simulink model "QuadRotor_PID_Simulink3d"  (R2014a)
settings: Solver=ode45  StartTime=0.0  StopTime=inf
PreLoadFcn:
  | load CommandsBus
model workspace (MAT data in the model file):
  MCOS : class17 (value not decoded)
  MCOS : class17 (value not decoded)
undefined symbols (not defined in the file or in its folder): X, Y, Z
libraries: sm_lib x829, nesl_utility x156, simulink x12, fl_lib x4, vrlib x4, aerolibtransform2 x1
(part 15 of 18)

== system QuadRotor_PID_Simulink3d/quadSimulation/Plant_Quad_Base/Quad_Yaw_Altitude/QuadRotor/P2/MotorA ==
  SpdMotor : Inport
  External Force and Torque : sm_lib/Forces and Torques/External Force and Torque  ForceResolutionFrame=AttachedFrame  EnableForceX=off  EnableForceY=off  EnableForceZ=on  EnableForce=off  TorqueResolutionFrame=AttachedFrame  EnableTorqueX=off  EnableTorqueY=off  EnableTorqueZ=on  EnableTorque=off  BlockFunction=simmechanics.library.forces_torques.external_force_torque
  Helice_1_RIGID : Subsystem
  PS-Simulink Converter : nesl_utility/PS-Simulink Converter  PhysicalDomain=network_engine_domain  SubClassName=ps_output  LeftPortType=input  RightPortType=output  PseudoPeriodic=off  Frequencies=[]  Unit=1  AffineConversion=off
  ReferenceFrame : sm_lib/Frames and Transforms/Reference Frame  BlockFunction=simmechanics.library.frames_transforms.reference_frame
  RevPropeller : sm_lib/Joints/Revolute Joint  SenseConstraintForce=off  SenseConstraintForceX=off  SenseConstraintForceY=off  SenseConstraintForceZ=off  SenseConstraintTorque=off  SenseConstraintTorqueX=off  SenseConstraintTorqueY=off  SenseConstraintTorqueZ=off  SenseTotalForce=off  SenseTotalForceX=off  SenseTotalForceY=off  SenseTotalForceZ=off  SenseTotalTorque=off  SenseTotalTorqueX=off  SenseTotalTorqueY=off  SenseTotalTorqueZ=off  CompositeWrenchDir=FollowerOnBase  CompositeWrenchFrame=BaseFrame  EquilibriumPosition=0  EquilibriumPositionUnits=rad  SpringStiffness=0  SpringStiffnessUnits=m*N/rad  DampingCoefficient=0  DampingCoefficientUnits=m*s*N/rad  TorqueActuationMode=InputTorque  MotionActuationMode=ComputedMotion  SensePosition=off  SenseVelocity=on  SenseAcceleration=off  SenseTorqueForce=off  PositionTargetValue=-56.842386520865752  PositionTargetValueUnits=deg  PositionTargetSpecify=off  PositionTargetPriority=Low  VelocityTargetValue=0  VelocityTargetValueUnits=deg/s  VelocityTargetSpecify=off  VelocityTargetPriority=High  BlockFunction=simmechanics.library.joints.revolute_joint
  Simulink-PS Converter : nesl_utility/Simulink-PS Converter  PhysicalDomain=network_engine_domain  SubClassName=ps_input  LeftPortType=input  RightPortType=output  PseudoPeriodic=off  Frequencies=[]  NoiseDistribution=none  NoiseParameters=[]  Unit=1  AffineConversion=off  InputFiltering=off  SimscapeFilterOrder=1  InputFilterTimeConstant=0.001  UdotUserProvided=1
  Simulink-PS Converter2 : nesl_utility/Simulink-PS Converter  PhysicalDomain=network_engine_domain  SubClassName=ps_input  LeftPortType=input  RightPortType=output  PseudoPeriodic=off  Frequencies=[]  NoiseDistribution=none  NoiseParameters=[]  Unit=1  AffineConversion=off  InputFiltering=off  SimscapeFilterOrder=1  InputFilterTimeConstant=0.001  UdotUserProvided=1
  Simulink-PS Converter3 : nesl_utility/Simulink-PS Converter  PhysicalDomain=network_engine_domain  SubClassName=ps_input  LeftPortType=input  RightPortType=output  PseudoPeriodic=off  Frequencies=[]  NoiseDistribution=none  NoiseParameters=[]  Unit=1  AffineConversion=off  InputFiltering=off  SimscapeFilterOrder=1  InputFilterTimeConstant=0.001  UdotUserProvided=1
  Thrust : MATLAB Function  TreatAsAtomicUnit=on
  Transform : sm_lib/Frames and Transforms/Rigid Transform  TranslationMethod=None  TranslationLengthUnit=m  TranslationStandardAxis=+Z  TranslationStandardOffset=0  TranslationCartesianOffset=[0 0 0]  TranslationROffset=0  TranslationROffsetUnits=m  TranslationZOffset=0  TranslationZOffsetUnits=m  TranslationThetaOffset=0  TranslationThetaOffsetUnits=deg  RotationMethod=None  RotationAngleUnits=deg  RotationStandardAxis=+Z  RotationAngle=0  RotationArbitraryAxis=[0 0 1]  FollAlignAxisA=+X  BaseAlignAxisA=+Y  FollAlignAxisB=+Y  BaseAlignAxisB=+Z  BlockFunction=simmechanics.library.frames_transforms.rigid_transform
  Transform1 : sm_lib/Frames and Transforms/Rigid Transform  TranslationMethod=Cartesian  TranslationLengthUnit=mm  TranslationStandardAxis=+Z  TranslationStandardOffset=0  TranslationCartesianOffset=[0 25 0]  TranslationROffset=0  TranslationROffsetUnits=m  TranslationZOffset=0  TranslationZOffsetUnits=m  TranslationThetaOffset=0  TranslationThetaOffsetUnits=deg  RotationMethod=ArbitraryAxis  RotationAngleUnits=rad  RotationStandardAxis=+Z  RotationAngle=1.6523019578475986  RotationArbitraryAxis=[-0.92164420581175521 -0.27438290571172536 -0.27438290571172536]  FollAlignAxisA=+X  BaseAlignAxisA=+Y  FollAlignAxisB=+Y  BaseAlignAxisB=+Z  BlockFunction=simmechanics.library.frames_transforms.rigid_transform
  Transform2 : sm_lib/Frames and Transforms/Rigid Transform  TranslationMethod=Cartesian  TranslationLengthUnit=mm  TranslationStandardAxis=+Z  TranslationStandardOffset=0  TranslationCartesianOffset=[-72.267600000000002 2.84903 0]  TranslationROffset=0  TranslationROffsetUnits=m  TranslationZOffset=0  TranslationZOffsetUnits=m  TranslationThetaOffset=0  TranslationThetaOffsetUnits=deg  RotationMethod=ArbitraryAxis  RotationAngleUnits=rad  RotationStandardAxis=+Z  RotationAngle=0.79748424782509497  RotationArbitraryAxis=[0 1 0]  FollAlignAxisA=+X  BaseAlignAxisA=+Y  FollAlignAxisB=+Y  BaseAlignAxisB=+Z  BlockFunction=simmechanics.library.frames_transforms.rigid_transform
  thrustRevoSpeedConstant : Constant  Value=thrustConstant
  thrustRevoSpeedConstant1 : Constant  Value=torqueConstant
  x18_11_2000kv_Micro_Brushless_1_RIGID : Subsystem
  F : PMIOPort  Port=1  Side=Left
  ThrustDebug : Outport
  wires:
  SpdMotor/1 -> Simulink-PS Converter/1
  thrustRevoSpeedConstant/1 -> Thrust/2(revCnst)
  PS-Simulink Converter/1 -> Thrust/1(revSpeed)
  thrustRevoSpeedConstant1/1 -> Thrust/3(revTqCnst)
  Thrust/2(Torque) -> Simulink-PS Converter3/1
  Thrust/1(Thrust) -> ThrustDebug/1, Simulink-PS Converter2/1
  connections:
  Transform/RConn1 -- x18_11_2000kv_Micro_Brushless_1_RIGID/LConn1
  Transform/LConn1 -- ReferenceFrame/RConn1 -- Transform2/RConn1 -- Transform1/LConn1
  Transform2/LConn1 -- F/RConn1
  External Force and Torque/RConn1 -- Helice_1_RIGID/LConn1 -- RevPropeller/RConn1
  RevPropeller/RConn2 -- PS-Simulink Converter/LConn1
  Simulink-PS Converter/RConn1 -- RevPropeller/LConn2
  Simulink-PS Converter3/RConn1 -- External Force and Torque/LConn2
  Simulink-PS Converter2/RConn1 -- External Force and Torque/LConn1
  Transform1/RConn1 -- RevPropeller/LConn1

== system QuadRotor_PID_Simulink3d/quadSimulation/Plant_Quad_Base/Quad_Yaw_Altitude/QuadRotor/P2/PernaInferior_1_RIGID ==
  ReferenceFrame : sm_lib/Frames and Transforms/Reference Frame  BlockFunction=simmechanics.library.frames_transforms.reference_frame
  Solid : sm_lib/Body Elements/Solid  InertiaType=Custom  Mass=0.0018417900000000001  MassUnits=kg  CenterOfMass=[-73.425399999999996 0 0.00026724000000000002]  CenterOfMassUnits=mm  MomentsOfInertia=[0.11792 1.59626 1.4790299999999998]  MomentsOfInertiaUnits=kg*mm^2  ProductsOfInertia=[0 -1.10078e-05 0]  ProductsOfInertiaUnits=kg*mm^2  DensityBased=on  Density=1000  DensityUnits=kg/(m^3)  GraphicType=FromGeometry  MarkerShape=Sphere  MarkerSize=10  MarkerSizeUnits=m  GraphicVisPropType=SimpleVisualProperties  GraphicDiffuseColor=[0.721569 0.54902 0.32]  GraphicSpecularColor=[0.5 0.5 0.5 1.0]  GraphicAmbientColor=[0.15 0.15 0.15 1.0]  GraphicEmissiveColor=[0.0 0.0 0.0 1.0]  GraphicShininess=75  GraphicOpacity=1  GeometryShape=FromFile  RectangleSize=[1 1]  RectangleSizeUnits=m  BrickDimensions=[1 1 1]  BrickDimensionUnits=m  CylinderRadius=1  CylinderRadiusUnits=m  CylinderLength=1  CylinderLengthUnits=m  SphereRadius=1  SphereRadiusUnits=m  EllipsoidRadii=[1 1 1]  EllipsoidRadiiUnits=m  ExtrusionCrossSection=[1 1; -1 1; -1 -1; 1 -1]  ExtrusionCrossSectionUnits=m  ExtrusionLength=1  ExtrusionLengthUnits=m  PolygonNumSides=3  PolygonOuterRadius=1  PolygonOuterRadiusUnits=m  ExtGeomFileType=STL  ExtGeomFileName=PernaInferior_Valor predeterminado_sldprt.STL  ExtGeomFileUnits=mm  RevolutionCrossSection=[1 1; 1 -1; 2 -1; 2 1]  RevolutionCrossSectionUnits=m  RevolutionExtent=Full  RevolutionAngle=180  RevolutionAngleUnits=deg  BlockFunction=simmechanics.library.body_elements.solid
  F : PMIOPort  Port=1  Side=Left
  connections:
  Solid/RConn1 -- ReferenceFrame/RConn1 -- F/RConn1

== system QuadRotor_PID_Simulink3d/quadSimulation/Plant_Quad_Base/Quad_Yaw_Altitude/QuadRotor/P2/PernaSuperior_1_RIGID ==
  ReferenceFrame : sm_lib/Frames and Transforms/Reference Frame  BlockFunction=simmechanics.library.frames_transforms.reference_frame
  Solid : sm_lib/Body Elements/Solid  InertiaType=Custom  Mass=0.0027502  MassUnits=kg  CenterOfMass=[-65.820400000000006 2.5968000000000004 -0.0043371999999999994]  CenterOfMassUnits=mm  MomentsOfInertia=[0.31065799999999999 2.3284099999999999 2.08405]  MomentsOfInertiaUnits=kg*mm^2  ProductsOfInertia=[-4.0442000000000003e-05 0.000357482 -0.0022943199999999999]  ProductsOfInertiaUnits=kg*mm^2  DensityBased=on  Density=1000  DensityUnits=kg/(m^3)  GraphicType=FromGeometry  MarkerShape=Sphere  MarkerSize=10  MarkerSizeUnits=m  GraphicVisPropType=SimpleVisualProperties  GraphicDiffuseColor=[0.721569 0.54902 0.32]  GraphicSpecularColor=[0.5 0.5 0.5 1.0]  GraphicAmbientColor=[0.15 0.15 0.15 1.0]  GraphicEmissiveColor=[0.0 0.0 0.0 1.0]  GraphicShininess=75  GraphicOpacity=1  GeometryShape=FromFile  RectangleSize=[1 1]  RectangleSizeUnits=m  BrickDimensions=[1 1 1]  BrickDimensionUnits=m  CylinderRadius=1  CylinderRadiusUnits=m  CylinderLength=1  CylinderLengthUnits=m  SphereRadius=1  SphereRadiusUnits=m  EllipsoidRadii=[1 1 1]  EllipsoidRadiiUnits=m  ExtrusionCrossSection=[1 1; -1 1; -1 -1; 1 -1]  ExtrusionCrossSectionUnits=m  ExtrusionLength=1  ExtrusionLengthUnits=m  PolygonNumSides=3  PolygonOuterRadius=1  PolygonOuterRadiusUnits=m  ExtGeomFileType=STL  ExtGeomFileName=PernaSuperior_Valor predeterminado_sldprt.STL  ExtGeomFileUnits=mm  RevolutionCrossSection=[1 1; 1 -1; 2 -1; 2 1]  RevolutionCrossSectionUnits=m  RevolutionExtent=Full  RevolutionAngle=180  RevolutionAngleUnits=deg  BlockFunction=simmechanics.library.body_elements.solid
  F : PMIOPort  Port=1  Side=Left
  connections:
  Solid/RConn1 -- ReferenceFrame/RConn1 -- F/RConn1

== system QuadRotor_PID_Simulink3d/quadSimulation/Plant_Quad_Base/Quad_Yaw_Altitude/QuadRotor/P3/MotorC ==
  SpdMotor : Inport
  External Force and Torque : sm_lib/Forces and Torques/External Force and Torque  ForceResolutionFrame=AttachedFrame  EnableForceX=off  EnableForceY=off  EnableForceZ=on  EnableForce=off  TorqueResolutionFrame=AttachedFrame  EnableTorqueX=off  EnableTorqueY=off  EnableTorqueZ=on  EnableTorque=off  BlockFunction=simmechanics.library.forces_torques.external_force_torque
  Helice_1_RIGID : Subsystem
  PS-Simulink Converter : nesl_utility/PS-Simulink Converter  PhysicalDomain=network_engine_domain  SubClassName=ps_output  LeftPortType=input  RightPortType=output  PseudoPeriodic=off  Frequencies=[]  Unit=1  AffineConversion=off
  ReferenceFrame : sm_lib/Frames and Transforms/Reference Frame  BlockFunction=simmechanics.library.frames_transforms.reference_frame
  RevPropeller : sm_lib/Joints/Revolute Joint  SenseConstraintForce=off  SenseConstraintForceX=off  SenseConstraintForceY=off  SenseConstraintForceZ=off  SenseConstraintTorque=off  SenseConstraintTorqueX=off  SenseConstraintTorqueY=off  SenseConstraintTorqueZ=off  SenseTotalForce=off  SenseTotalForceX=off  SenseTotalForceY=off  SenseTotalForceZ=off  SenseTotalTorque=off  SenseTotalTorqueX=off  SenseTotalTorqueY=off  SenseTotalTorqueZ=off  CompositeWrenchDir=FollowerOnBase  CompositeWrenchFrame=BaseFrame  EquilibriumPosition=0  EquilibriumPositionUnits=rad  SpringStiffness=0  SpringStiffnessUnits=m*N/rad  DampingCoefficient=0  DampingCoefficientUnits=m*s*N/rad  TorqueActuationMode=InputTorque  MotionActuationMode=ComputedMotion  SensePosition=off  SenseVelocity=on  SenseAcceleration=off  SenseTorqueForce=off  PositionTargetValue=-56.842386520865752  PositionTargetValueUnits=deg  PositionTargetSpecify=off  PositionTargetPriority=Low  VelocityTargetValue=0  VelocityTargetValueUnits=deg/s  VelocityTargetSpecify=off  VelocityTargetPriority=High  BlockFunction=simmechanics.library.joints.revolute_joint
  Simulink-PS Converter : nesl_utility/Simulink-PS Converter  PhysicalDomain=network_engine_domain  SubClassName=ps_input  LeftPortType=input  RightPortType=output  PseudoPeriodic=off  Frequencies=[]  NoiseDistribution=none  NoiseParameters=[]  Unit=1  AffineConversion=off  InputFiltering=off  SimscapeFilterOrder=1  InputFilterTimeConstant=0.001  UdotUserProvided=1
  Simulink-PS Converter2 : nesl_utility/Simulink-PS Converter  PhysicalDomain=network_engine_domain  SubClassName=ps_input  LeftPortType=input  RightPortType=output  PseudoPeriodic=off  Frequencies=[]  NoiseDistribution=none  NoiseParameters=[]  Unit=1  AffineConversion=off  InputFiltering=off  SimscapeFilterOrder=1  InputFilterTimeConstant=0.001  UdotUserProvided=1
  Simulink-PS Converter3 : nesl_utility/Simulink-PS Converter  PhysicalDomain=network_engine_domain  SubClassName=ps_input  LeftPortType=input  RightPortType=output  PseudoPeriodic=off  Frequencies=[]  NoiseDistribution=none  NoiseParameters=[]  Unit=1  AffineConversion=off  InputFiltering=off  SimscapeFilterOrder=1  InputFilterTimeConstant=0.001  UdotUserProvided=1
  Thrust : MATLAB Function  TreatAsAtomicUnit=on
  Transform : sm_lib/Frames and Transforms/Rigid Transform  TranslationMethod=None  TranslationLengthUnit=m  TranslationStandardAxis=+Z  TranslationStandardOffset=0  TranslationCartesianOffset=[0 0 0]  TranslationROffset=0  TranslationROffsetUnits=m  TranslationZOffset=0  TranslationZOffsetUnits=m  TranslationThetaOffset=0  TranslationThetaOffsetUnits=deg  RotationMethod=None  RotationAngleUnits=deg  RotationStandardAxis=+Z  RotationAngle=0  RotationArbitraryAxis=[0 0 1]  FollAlignAxisA=+X  BaseAlignAxisA=+Y  FollAlignAxisB=+Y  BaseAlignAxisB=+Z  BlockFunction=simmechanics.library.frames_transforms.rigid_transform
  Transform1 : sm_lib/Frames and Transforms/Rigid Transform  TranslationMethod=Cartesian  TranslationLengthUnit=mm  TranslationStandardAxis=+Z  TranslationStandardOffset=0  TranslationCartesianOffset=[0 25 0]  TranslationROffset=0  TranslationROffsetUnits=m  TranslationZOffset=0  TranslationZOffsetUnits=m  TranslationThetaOffset=0  TranslationThetaOffsetUnits=deg  RotationMethod=ArbitraryAxis  RotationAngleUnits=rad  RotationStandardAxis=+Z  RotationAngle=1.6523019578475986  RotationArbitraryAxis=[-0.92164420581175521 -0.27438290571172536 -0.27438290571172536]  FollAlignAxisA=+X  BaseAlignAxisA=+Y  FollAlignAxisB=+Y  BaseAlignAxisB=+Z  BlockFunction=simmechanics.library.frames_transforms.rigid_transform
  Transform2 : sm_lib/Frames and Transforms/Rigid Transform  TranslationMethod=Cartesian  TranslationLengthUnit=mm  TranslationStandardAxis=+Z  TranslationStandardOffset=0  TranslationCartesianOffset=[-72.267600000000002 2.84903 0]  TranslationROffset=0  TranslationROffsetUnits=m  TranslationZOffset=0  TranslationZOffsetUnits=m  TranslationThetaOffset=0  TranslationThetaOffsetUnits=deg  RotationMethod=ArbitraryAxis  RotationAngleUnits=rad  RotationStandardAxis=+Z  RotationAngle=0.79748424782509497  RotationArbitraryAxis=[0 1 0]  FollAlignAxisA=+X  BaseAlignAxisA=+Y  FollAlignAxisB=+Y  BaseAlignAxisB=+Z  BlockFunction=simmechanics.library.frames_transforms.rigid_transform
  thrustRevoSpeedConstant : Constant  Value=thrustConstant
  thrustRevoSpeedConstant1 : Constant  Value=torqueConstant
  x18_11_2000kv_Micro_Brushless_1_RIGID : Subsystem
  F : PMIOPort  Port=1  Side=Left
  ThrustDebug : Outport
  wires:
  SpdMotor/1 -> Simulink-PS Converter/1
  thrustRevoSpeedConstant/1 -> Thrust/2(revCnst)
  PS-Simulink Converter/1 -> Thrust/1(revSpeed)
  thrustRevoSpeedConstant1/1 -> Thrust/3(revTqCnst)
  Thrust/2(Torque) -> Simulink-PS Converter3/1
  Thrust/1(Thrust) -> ThrustDebug/1, Simulink-PS Converter2/1
  connections:
  Transform/RConn1 -- x18_11_2000kv_Micro_Brushless_1_RIGID/LConn1
  ReferenceFrame/RConn1 -- Transform/LConn1 -- Transform2/RConn1 -- Transform1/LConn1
  Transform2/LConn1 -- F/RConn1
  External Force and Torque/RConn1 -- Helice_1_RIGID/LConn1 -- RevPropeller/RConn1
  RevPropeller/RConn2 -- PS-Simulink Converter/LConn1
  Simulink-PS Converter3/RConn1 -- External Force and Torque/LConn2
  Simulink-PS Converter2/RConn1 -- External Force and Torque/LConn1
  Simulink-PS Converter/RConn1 -- RevPropeller/LConn2
  Transform1/RConn1 -- RevPropeller/LConn1

== system QuadRotor_PID_Simulink3d/quadSimulation/Plant_Quad_Base/Quad_Yaw_Altitude/QuadRotor/P3/PernaInferior_1_RIGID ==
  ReferenceFrame : sm_lib/Frames and Transforms/Reference Frame  BlockFunction=simmechanics.library.frames_transforms.reference_frame
  Solid : sm_lib/Body Elements/Solid  InertiaType=Custom  Mass=0.0018417900000000001  MassUnits=kg  CenterOfMass=[-73.425399999999996 0 0.00026724000000000002]  CenterOfMassUnits=mm  MomentsOfInertia=[0.11792 1.59626 1.4790299999999998]  MomentsOfInertiaUnits=kg*mm^2  ProductsOfInertia=[0 -1.10078e-05 0]  ProductsOfInertiaUnits=kg*mm^2  DensityBased=on  Density=1000  DensityUnits=kg/(m^3)  GraphicType=FromGeometry  MarkerShape=Sphere  MarkerSize=10  MarkerSizeUnits=m  GraphicVisPropType=SimpleVisualProperties  GraphicDiffuseColor=[0.721569 0.54902 0.32]  GraphicSpecularColor=[0.5 0.5 0.5 1.0]  GraphicAmbientColor=[0.15 0.15 0.15 1.0]  GraphicEmissiveColor=[0.0 0.0 0.0 1.0]  GraphicShininess=75  GraphicOpacity=1  GeometryShape=FromFile  RectangleSize=[1 1]  RectangleSizeUnits=m  BrickDimensions=[1 1 1]  BrickDimensionUnits=m  CylinderRadius=1  CylinderRadiusUnits=m  CylinderLength=1  CylinderLengthUnits=m  SphereRadius=1  SphereRadiusUnits=m  EllipsoidRadii=[1 1 1]  EllipsoidRadiiUnits=m  ExtrusionCrossSection=[1 1; -1 1; -1 -1; 1 -1]  ExtrusionCrossSectionUnits=m  ExtrusionLength=1  ExtrusionLengthUnits=m  PolygonNumSides=3  PolygonOuterRadius=1  PolygonOuterRadiusUnits=m  ExtGeomFileType=STL  ExtGeomFileName=PernaInferior_Valor predeterminado_sldprt.STL  ExtGeomFileUnits=mm  RevolutionCrossSection=[1 1; 1 -1; 2 -1; 2 1]  RevolutionCrossSectionUnits=m  RevolutionExtent=Full  RevolutionAngle=180  RevolutionAngleUnits=deg  BlockFunction=simmechanics.library.body_elements.solid
  F : PMIOPort  Port=1  Side=Left
  connections:
  Solid/RConn1 -- ReferenceFrame/RConn1 -- F/RConn1

== system QuadRotor_PID_Simulink3d/quadSimulation/Plant_Quad_Base/Quad_Yaw_Altitude/QuadRotor/P3/PernaSuperior_1_RIGID ==
  ReferenceFrame : sm_lib/Frames and Transforms/Reference Frame  BlockFunction=simmechanics.library.frames_transforms.reference_frame
  Solid : sm_lib/Body Elements/Solid  InertiaType=Custom  Mass=0.0027502  MassUnits=kg  CenterOfMass=[-65.820400000000006 2.5968000000000004 -0.0043371999999999994]  CenterOfMassUnits=mm  MomentsOfInertia=[0.31065799999999999 2.3284099999999999 2.08405]  MomentsOfInertiaUnits=kg*mm^2  ProductsOfInertia=[-4.0442000000000003e-05 0.000357482 -0.0022943199999999999]  ProductsOfInertiaUnits=kg*mm^2  DensityBased=on  Density=1000  DensityUnits=kg/(m^3)  GraphicType=FromGeometry  MarkerShape=Sphere  MarkerSize=10  MarkerSizeUnits=m  GraphicVisPropType=SimpleVisualProperties  GraphicDiffuseColor=[0.721569 0.54902 0.32]  GraphicSpecularColor=[0.5 0.5 0.5 1.0]  GraphicAmbientColor=[0.15 0.15 0.15 1.0]  GraphicEmissiveColor=[0.0 0.0 0.0 1.0]  GraphicShininess=75  GraphicOpacity=1  GeometryShape=FromFile  RectangleSize=[1 1]  RectangleSizeUnits=m  BrickDimensions=[1 1 1]  BrickDimensionUnits=m  CylinderRadius=1  CylinderRadiusUnits=m  CylinderLength=1  CylinderLengthUnits=m  SphereRadius=1  SphereRadiusUnits=m  EllipsoidRadii=[1 1 1]  EllipsoidRadiiUnits=m  ExtrusionCrossSection=[1 1; -1 1; -1 -1; 1 -1]  ExtrusionCrossSectionUnits=m  ExtrusionLength=1  ExtrusionLengthUnits=m  PolygonNumSides=3  PolygonOuterRadius=1  PolygonOuterRadiusUnits=m  ExtGeomFileType=STL  ExtGeomFileName=PernaSuperior_Valor predeterminado_sldprt.STL  ExtGeomFileUnits=mm  RevolutionCrossSection=[1 1; 1 -1; 2 -1; 2 1]  RevolutionCrossSectionUnits=m  RevolutionExtent=Full  RevolutionAngle=180  RevolutionAngleUnits=deg  BlockFunction=simmechanics.library.body_elements.solid
  F : PMIOPort  Port=1  Side=Left
  connections:
  Solid/RConn1 -- ReferenceFrame/RConn1 -- F/RConn1

== system QuadRotor_PID_Simulink3d/quadSimulation/Plant_Quad_Base/Quad_Yaw_Altitude/QuadRotor/P4/MotorD ==
  SpdMotor : Inport
  External Force and Torque : sm_lib/Forces and Torques/External Force and Torque  ForceResolutionFrame=AttachedFrame  EnableForceX=off  EnableForceY=off  EnableForceZ=on  EnableForce=off  TorqueResolutionFrame=AttachedFrame  EnableTorqueX=off  EnableTorqueY=off  EnableTorqueZ=on  EnableTorque=off  BlockFunction=simmechanics.library.forces_torques.external_force_torque
  Helice_1_RIGID : Subsystem
  PS-Simulink Converter : nesl_utility/PS-Simulink Converter  PhysicalDomain=network_engine_domain  SubClassName=ps_output  LeftPortType=input  RightPortType=output  PseudoPeriodic=off  Frequencies=[]  Unit=1  AffineConversion=off
  ReferenceFrame : sm_lib/Frames and Transforms/Reference Frame  BlockFunction=simmechanics.library.frames_transforms.reference_frame
  RevPropeller : sm_lib/Joints/Revolute Joint  SenseConstraintForce=off  SenseConstraintForceX=off  SenseConstraintForceY=off  SenseConstraintForceZ=off  SenseConstraintTorque=off  SenseConstraintTorqueX=off  SenseConstraintTorqueY=off  SenseConstraintTorqueZ=off  SenseTotalForce=off  SenseTotalForceX=off  SenseTotalForceY=off  SenseTotalForceZ=off  SenseTotalTorque=off  SenseTotalTorqueX=off  SenseTotalTorqueY=off  SenseTotalTorqueZ=off  CompositeWrenchDir=FollowerOnBase  CompositeWrenchFrame=BaseFrame  EquilibriumPosition=0  EquilibriumPositionUnits=rad  SpringStiffness=0  SpringStiffnessUnits=m*N/rad  DampingCoefficient=0  DampingCoefficientUnits=m*s*N/rad  TorqueActuationMode=InputTorque  MotionActuationMode=ComputedMotion  SensePosition=off  SenseVelocity=on  SenseAcceleration=off  SenseTorqueForce=off  PositionTargetValue=-56.842386520865752  PositionTargetValueUnits=deg  PositionTargetSpecify=off  PositionTargetPriority=Low  VelocityTargetValue=0  VelocityTargetValueUnits=deg/s  VelocityTargetSpecify=off  VelocityTargetPriority=High  BlockFunction=simmechanics.library.joints.revolute_joint
  Simulink-PS Converter : nesl_utility/Simulink-PS Converter  PhysicalDomain=network_engine_domain  SubClassName=ps_input  LeftPortType=input  RightPortType=output  PseudoPeriodic=off  Frequencies=[]  NoiseDistribution=none  NoiseParameters=[]  Unit=1  AffineConversion=off  InputFiltering=off  SimscapeFilterOrder=1  InputFilterTimeConstant=0.001  UdotUserProvided=1
  Simulink-PS Converter2 : nesl_utility/Simulink-PS Converter  PhysicalDomain=network_engine_domain  SubClassName=ps_input  LeftPortType=input  RightPortType=output  PseudoPeriodic=off  Frequencies=[]  NoiseDistribution=none  NoiseParameters=[]  Unit=1  AffineConversion=off  InputFiltering=off  SimscapeFilterOrder=1  InputFilterTimeConstant=0.001  UdotUserProvided=1
  Simulink-PS Converter3 : nesl_utility/Simulink-PS Converter  PhysicalDomain=network_engine_domain  SubClassName=ps_input  LeftPortType=input  RightPortType=output  PseudoPeriodic=off  Frequencies=[]  NoiseDistribution=none  NoiseParameters=[]  Unit=1  AffineConversion=off  InputFiltering=off  SimscapeFilterOrder=1  InputFilterTimeConstant=0.001  UdotUserProvided=1
  Thrust : MATLAB Function  TreatAsAtomicUnit=on
  Transform : sm_lib/Frames and Transforms/Rigid Transform  TranslationMethod=None  TranslationLengthUnit=m  TranslationStandardAxis=+Z  TranslationStandardOffset=0  TranslationCartesianOffset=[0 0 0]  TranslationROffset=0  TranslationROffsetUnits=m  TranslationZOffset=0  TranslationZOffsetUnits=m  TranslationThetaOffset=0  TranslationThetaOffsetUnits=deg  RotationMethod=None  RotationAngleUnits=deg  RotationStandardAxis=+Z  RotationAngle=0  RotationArbitraryAxis=[0 0 1]  FollAlignAxisA=+X  BaseAlignAxisA=+Y  FollAlignAxisB=+Y  BaseAlignAxisB=+Z  BlockFunction=simmechanics.library.frames_transforms.rigid_transform
  Transform1 : sm_lib/Frames and Transforms/Rigid Transform  TranslationMethod=Cartesian  TranslationLengthUnit=mm  TranslationStandardAxis=+Z  TranslationStandardOffset=0  TranslationCartesianOffset=[0 25 0]  TranslationROffset=0  TranslationROffsetUnits=m  TranslationZOffset=0  TranslationZOffsetUnits=m  TranslationThetaOffset=0  TranslationThetaOffsetUnits=deg  RotationMethod=ArbitraryAxis  RotationAngleUnits=rad  RotationStandardAxis=+Z  RotationAngle=1.6523019578475986  RotationArbitraryAxis=[-0.92164420581175521 -0.27438290571172536 -0.27438290571172536]  FollAlignAxisA=+X  BaseAlignAxisA=+Y  FollAlignAxisB=+Y  BaseAlignAxisB=+Z  BlockFunction=simmechanics.library.frames_transforms.rigid_transform
  Transform2 : sm_lib/Frames and Transforms/Rigid Transform  TranslationMethod=Cartesian  TranslationLengthUnit=mm  TranslationStandardAxis=+Z  TranslationStandardOffset=0  TranslationCartesianOffset=[-72.267600000000002 2.84903 0]  TranslationROffset=0  TranslationROffsetUnits=m  TranslationZOffset=0  TranslationZOffsetUnits=m  TranslationThetaOffset=0  TranslationThetaOffsetUnits=deg  RotationMethod=ArbitraryAxis  RotationAngleUnits=rad  RotationStandardAxis=+Z  RotationAngle=0.79748424782509497  RotationArbitraryAxis=[0 1 0]  FollAlignAxisA=+X  BaseAlignAxisA=+Y  FollAlignAxisB=+Y  BaseAlignAxisB=+Z  BlockFunction=simmechanics.library.frames_transforms.rigid_transform
  thrustRevoSpeedConstant : Constant  Value=thrustConstant
  thrustRevoSpeedConstant1 : Constant  Value=torqueConstant
  x18_11_2000kv_Micro_Brushless_1_RIGID : Subsystem
  F : PMIOPort  Port=1  Side=Left
  ThrustDebug : Outport
  wires:
  SpdMotor/1 -> Simulink-PS Converter/1
  Thrust/1(Thrust) -> ThrustDebug/1, Simulink-PS Converter2/1
  thrustRevoSpeedConstant/1 -> Thrust/2(revCnst)
  PS-Simulink Converter/1 -> Thrust/1(revSpeed)
  thrustRevoSpeedConstant1/1 -> Thrust/3(revTqCnst)
  Thrust/2(Torque) -> Simulink-PS Converter3/1
  connections:
  Transform/RConn1 -- x18_11_2000kv_Micro_Brushless_1_RIGID/LConn1
  Transform/LConn1 -- ReferenceFrame/RConn1 -- Transform2/RConn1 -- Transform1/LConn1
  Transform2/LConn1 -- F/RConn1
  External Force and Torque/RConn1 -- Helice_1_RIGID/LConn1 -- RevPropeller/RConn1
  Simulink-PS Converter3/RConn1 -- External Force and Torque/LConn2
  Simulink-PS Converter2/RConn1 -- External Force and Torque/LConn1
  RevPropeller/RConn2 -- PS-Simulink Converter/LConn1
  Simulink-PS Converter/RConn1 -- RevPropeller/LConn2
  Transform1/RConn1 -- RevPropeller/LConn1

== system QuadRotor_PID_Simulink3d/quadSimulation/Plant_Quad_Base/Quad_Yaw_Altitude/QuadRotor/P4/PernaInferior_1_RIGID ==
  ReferenceFrame : sm_lib/Frames and Transforms/Reference Frame  BlockFunction=simmechanics.library.frames_transforms.reference_frame
  Solid : sm_lib/Body Elements/Solid  InertiaType=Custom  Mass=0.0018417900000000001  MassUnits=kg  CenterOfMass=[-73.425399999999996 0 0.00026724000000000002]  CenterOfMassUnits=mm  MomentsOfInertia=[0.11792 1.59626 1.4790299999999998]  MomentsOfInertiaUnits=kg*mm^2  ProductsOfInertia=[0 -1.10078e-05 0]  ProductsOfInertiaUnits=kg*mm^2  DensityBased=on  Density=1000  DensityUnits=kg/(m^3)  GraphicType=FromGeometry  MarkerShape=Sphere  MarkerSize=10  MarkerSizeUnits=m  GraphicVisPropType=SimpleVisualProperties  GraphicDiffuseColor=[0.721569 0.54902 0.32]  GraphicSpecularColor=[0.5 0.5 0.5 1.0]  GraphicAmbientColor=[0.15 0.15 0.15 1.0]  GraphicEmissiveColor=[0.0 0.0 0.0 1.0]  GraphicShininess=75  GraphicOpacity=1  GeometryShape=FromFile  RectangleSize=[1 1]  RectangleSizeUnits=m  BrickDimensions=[1 1 1]  BrickDimensionUnits=m  CylinderRadius=1  CylinderRadiusUnits=m  CylinderLength=1  CylinderLengthUnits=m  SphereRadius=1  SphereRadiusUnits=m  EllipsoidRadii=[1 1 1]  EllipsoidRadiiUnits=m  ExtrusionCrossSection=[1 1; -1 1; -1 -1; 1 -1]  ExtrusionCrossSectionUnits=m  ExtrusionLength=1  ExtrusionLengthUnits=m  PolygonNumSides=3  PolygonOuterRadius=1  PolygonOuterRadiusUnits=m  ExtGeomFileType=STL  ExtGeomFileName=PernaInferior_Valor predeterminado_sldprt.STL  ExtGeomFileUnits=mm  RevolutionCrossSection=[1 1; 1 -1; 2 -1; 2 1]  RevolutionCrossSectionUnits=m  RevolutionExtent=Full  RevolutionAngle=180  RevolutionAngleUnits=deg  BlockFunction=simmechanics.library.body_elements.solid
  F : PMIOPort  Port=1  Side=Left
  connections:
  Solid/RConn1 -- ReferenceFrame/RConn1 -- F/RConn1

== system QuadRotor_PID_Simulink3d/quadSimulation/Plant_Quad_Base/Quad_Yaw_Altitude/QuadRotor/P4/PernaSuperior_1_RIGID ==
  ReferenceFrame : sm_lib/Frames and Transforms/Reference Frame  BlockFunction=simmechanics.library.frames_transforms.reference_frame
  Solid : sm_lib/Body Elements/Solid  InertiaType=Custom  Mass=0.0027502  MassUnits=kg  CenterOfMass=[-65.820400000000006 2.5968000000000004 -0.0043371999999999994]  CenterOfMassUnits=mm  MomentsOfInertia=[0.31065799999999999 2.3284099999999999 2.08405]  MomentsOfInertiaUnits=kg*mm^2  ProductsOfInertia=[-4.0442000000000003e-05 0.000357482 -0.0022943199999999999]  ProductsOfInertiaUnits=kg*mm^2  DensityBased=on  Density=1000  DensityUnits=kg/(m^3)  GraphicType=FromGeometry  MarkerShape=Sphere  MarkerSize=10  MarkerSizeUnits=m  GraphicVisPropType=SimpleVisualProperties  GraphicDiffuseColor=[0.721569 0.54902 0.32]  GraphicSpecularColor=[0.5 0.5 0.5 1.0]  GraphicAmbientColor=[0.15 0.15 0.15 1.0]  GraphicEmissiveColor=[0.0 0.0 0.0 1.0]  GraphicShininess=75  GraphicOpacity=1  GeometryShape=FromFile  RectangleSize=[1 1]  RectangleSizeUnits=m  BrickDimensions=[1 1 1]  BrickDimensionUnits=m  CylinderRadius=1  CylinderRadiusUnits=m  CylinderLength=1  CylinderLengthUnits=m  SphereRadius=1  SphereRadiusUnits=m  EllipsoidRadii=[1 1 1]  EllipsoidRadiiUnits=m  ExtrusionCrossSection=[1 1; -1 1; -1 -1; 1 -1]  ExtrusionCrossSectionUnits=m  ExtrusionLength=1  ExtrusionLengthUnits=m  PolygonNumSides=3  PolygonOuterRadius=1  PolygonOuterRadiusUnits=m  ExtGeomFileType=STL  ExtGeomFileName=PernaSuperior_Valor predeterminado_sldprt.STL  ExtGeomFileUnits=mm  RevolutionCrossSection=[1 1; 1 -1; 2 -1; 2 1]  RevolutionCrossSectionUnits=m  RevolutionExtent=Full  RevolutionAngle=180  RevolutionAngleUnits=deg  BlockFunction=simmechanics.library.body_elements.solid
  F : PMIOPort  Port=1  Side=Left
  connections:
  Solid/RConn1 -- ReferenceFrame/RConn1 -- F/RConn1

== system QuadRotor_PID_Simulink3d/quadSimulation/Plant_Quad_Base/Quad_6Dof/QuadRotor/P1/MotorB/Helice_1_RIGID ==
  ReferenceFrame : sm_lib/Frames and Transforms/Reference Frame  BlockFunction=simmechanics.library.frames_transforms.reference_frame
  Solid : sm_lib/Body Elements/Solid  InertiaType=Custom  Mass=0.00049709299999999999  MassUnits=kg  CenterOfMass=[0 0 -0.00012752400000000001]  CenterOfMassUnits=mm  MomentsOfInertia=[0.0011848399999999999 0.31476899999999997 0.31557499999999999]  MomentsOfInertiaUnits=kg*mm^2  ProductsOfInertia=[0 0 -7.1669699999999998e-06]  ProductsOfInertiaUnits=kg*mm^2  DensityBased=on  Density=1000  DensityUnits=kg/(m^3)  GraphicType=FromGeometry  MarkerShape=Sphere  MarkerSize=10  MarkerSizeUnits=m  GraphicVisPropType=SimpleVisualProperties  GraphicDiffuseColor=[1 1 1]  GraphicSpecularColor=[0.5 0.5 0.5 1.0]  GraphicAmbientColor=[0.15 0.15 0.15 1.0]  GraphicEmissiveColor=[0.0 0.0 0.0 1.0]  GraphicShininess=75  GraphicOpacity=1  GeometryShape=FromFile  RectangleSize=[1 1]  RectangleSizeUnits=m  BrickDimensions=[1 1 1]  BrickDimensionUnits=m  CylinderRadius=1  CylinderRadiusUnits=m  CylinderLength=1  CylinderLengthUnits=m  SphereRadius=1  SphereRadiusUnits=m  EllipsoidRadii=[1 1 1]  EllipsoidRadiiUnits=m  ExtrusionCrossSection=[1 1; -1 1; -1 -1; 1 -1]  ExtrusionCrossSectionUnits=m  ExtrusionLength=1  ExtrusionLengthUnits=m  PolygonNumSides=3  PolygonOuterRadius=1  PolygonOuterRadiusUnits=m  ExtGeomFileType=STL  ExtGeomFileName=Helice_Valor predeterminado_sldprt.STL  ExtGeomFileUnits=mm  RevolutionCrossSection=[1 1; 1 -1; 2 -1; 2 1]  RevolutionCrossSectionUnits=m  RevolutionExtent=Full  RevolutionAngle=180  RevolutionAngleUnits=deg  BlockFunction=simmechanics.library.body_elements.solid
  F : PMIOPort  Port=1  Side=Left
  connections:
  Solid/RConn1 -- ReferenceFrame/RConn1 -- F/RConn1

== system QuadRotor_PID_Simulink3d/quadSimulation/Plant_Quad_Base/Quad_6Dof/QuadRotor/P1/MotorB/x18_11_2000kv_Micro_Brushless_1_RIGID ==
  ReferenceFrame : sm_lib/Frames and Transforms/Reference Frame  BlockFunction=simmechanics.library.frames_transforms.reference_frame
  Solid : sm_lib/Body Elements/Solid  InertiaType=Custom  Mass=10  MassUnits=g  CenterOfMass=[0 12.8438 0]  CenterOfMassUnits=mm  MomentsOfInertia=[0.43731300000000001 0.28562900000000002 0.43731300000000001]  MomentsOfInertiaUnits=kg*mm^2  ProductsOfInertia=[0 0 0]  ProductsOfInertiaUnits=kg*mm^2  DensityBased=on  Density=1000  DensityUnits=kg/(m^3)  GraphicType=FromGeometry  MarkerShape=Sphere  MarkerSize=10  MarkerSizeUnits=m  GraphicVisPropType=SimpleVisualProperties  GraphicDiffuseColor=[0.894118 0.913725 0.929412]  GraphicSpecularColor=[0.5 0.5 0.5 1.0]  GraphicAmbientColor=[0.15 0.15 0.15 1.0]  GraphicEmissiveColor=[0.0 0.0 0.0 1.0]  GraphicShininess=75  GraphicOpacity=1  GeometryShape=FromFile  RectangleSize=[1 1]  RectangleSizeUnits=m  BrickDimensions=[1 1 1]  BrickDimensionUnits=m  CylinderRadius=1  CylinderRadiusUnits=m  CylinderLength=1  CylinderLengthUnits=m  SphereRadius=1  SphereRadiusUnits=m  EllipsoidRadii=[1 1 1]  EllipsoidRadiiUnits=m  ExtrusionCrossSection=[1 1; -1 1; -1 -1; 1 -1]  ExtrusionCrossSectionUnits=m  ExtrusionLength=1  ExtrusionLengthUnits=m  PolygonNumSides=3  PolygonOuterRadius=1  PolygonOuterRadiusUnits=m  ExtGeomFileType=STL  ExtGeomFileName=18-11 2000kv Micro Brushless_Valor predeterminado_sldprt.STL  ExtGeomFileUnits=mm  RevolutionCrossSection=[1 1; 1 -1; 2 -1; 2 1]  RevolutionCrossSectionUnits=m  RevolutionExtent=Full  RevolutionAngle=180  RevolutionAngleUnits=deg  BlockFunction=simmechanics.library.body_elements.solid
  F : PMIOPort  Port=1  Side=Left
  connections:
  Solid/RConn1 -- ReferenceFrame/RConn1 -- F/RConn1

== system QuadRotor_PID_Simulink3d/quadSimulation/Plant_Quad_Base/Quad_6Dof/QuadRotor/P2/MotorA/Helice_1_RIGID ==
  ReferenceFrame : sm_lib/Frames and Transforms/Reference Frame  BlockFunction=simmechanics.library.frames_transforms.reference_frame
  Solid : sm_lib/Body Elements/Solid  InertiaType=Custom  Mass=0.00049709299999999999  MassUnits=kg  CenterOfMass=[0 0 -0.00012752400000000001]  CenterOfMassUnits=mm  MomentsOfInertia=[0.0011848399999999999 0.31476899999999997 0.31557499999999999]  MomentsOfInertiaUnits=kg*mm^2  ProductsOfInertia=[0 0 -7.1669699999999998e-06]  ProductsOfInertiaUnits=kg*mm^2  DensityBased=on  Density=1000  DensityUnits=kg/(m^3)  GraphicType=FromGeometry  MarkerShape=Sphere  MarkerSize=10  MarkerSizeUnits=m  GraphicVisPropType=SimpleVisualProperties  GraphicDiffuseColor=[1 1 1]  GraphicSpecularColor=[0.5 0.5 0.5 1.0]  GraphicAmbientColor=[0.15 0.15 0.15 1.0]  GraphicEmissiveColor=[0.0 0.0 0.0 1.0]  GraphicShininess=75  GraphicOpacity=1  GeometryShape=FromFile  RectangleSize=[1 1]  RectangleSizeUnits=m  BrickDimensions=[1 1 1]  BrickDimensionUnits=m  CylinderRadius=1  CylinderRadiusUnits=m  CylinderLength=1  CylinderLengthUnits=m  SphereRadius=1  SphereRadiusUnits=m  EllipsoidRadii=[1 1 1]  EllipsoidRadiiUnits=m  ExtrusionCrossSection=[1 1; -1 1; -1 -1; 1 -1]  ExtrusionCrossSectionUnits=m  ExtrusionLength=1  ExtrusionLengthUnits=m  PolygonNumSides=3  PolygonOuterRadius=1  PolygonOuterRadiusUnits=m  ExtGeomFileType=STL  ExtGeomFileName=Helice_Valor predeterminado_sldprt.STL  ExtGeomFileUnits=mm  RevolutionCrossSection=[1 1; 1 -1; 2 -1; 2 1]  RevolutionCrossSectionUnits=m  RevolutionExtent=Full  RevolutionAngle=180  RevolutionAngleUnits=deg  BlockFunction=simmechanics.library.body_elements.solid
  F : PMIOPort  Port=1  Side=Left
  connections:
  Solid/RConn1 -- ReferenceFrame/RConn1 -- F/RConn1

== system QuadRotor_PID_Simulink3d/quadSimulation/Plant_Quad_Base/Quad_6Dof/QuadRotor/P2/MotorA/x18_11_2000kv_Micro_Brushless_1_RIGID ==
  ReferenceFrame : sm_lib/Frames and Transforms/Reference Frame  BlockFunction=simmechanics.library.frames_transforms.reference_frame
  Solid : sm_lib/Body Elements/Solid  InertiaType=Custom  Mass=10  MassUnits=g  CenterOfMass=[0 12.8438 0]  CenterOfMassUnits=mm  MomentsOfInertia=[0.43731300000000001 0.28562900000000002 0.43731300000000001]  MomentsOfInertiaUnits=kg*mm^2  ProductsOfInertia=[0 0 0]  ProductsOfInertiaUnits=kg*mm^2  DensityBased=on  Density=1000  DensityUnits=kg/(m^3)  GraphicType=FromGeometry  MarkerShape=Sphere  MarkerSize=10  MarkerSizeUnits=m  GraphicVisPropType=SimpleVisualProperties  GraphicDiffuseColor=[0.894118 0.913725 0.929412]  GraphicSpecularColor=[0.5 0.5 0.5 1.0]  GraphicAmbientColor=[0.15 0.15 0.15 1.0]  GraphicEmissiveColor=[0.0 0.0 0.0 1.0]  GraphicShininess=75  GraphicOpacity=1  GeometryShape=FromFile  RectangleSize=[1 1]  RectangleSizeUnits=m  BrickDimensions=[1 1 1]  BrickDimensionUnits=m  CylinderRadius=1  CylinderRadiusUnits=m  CylinderLength=1  CylinderLengthUnits=m  SphereRadius=1  SphereRadiusUnits=m  EllipsoidRadii=[1 1 1]  EllipsoidRadiiUnits=m  ExtrusionCrossSection=[1 1; -1 1; -1 -1; 1 -1]  ExtrusionCrossSectionUnits=m  ExtrusionLength=1  ExtrusionLengthUnits=m  PolygonNumSides=3  PolygonOuterRadius=1  PolygonOuterRadiusUnits=m  ExtGeomFileType=STL  ExtGeomFileName=18-11 2000kv Micro Brushless_Valor predeterminado_sldprt.STL  ExtGeomFileUnits=mm  RevolutionCrossSection=[1 1; 1 -1; 2 -1; 2 1]  RevolutionCrossSectionUnits=m  RevolutionExtent=Full  RevolutionAngle=180  RevolutionAngleUnits=deg  BlockFunction=simmechanics.library.body_elements.solid
  F : PMIOPort  Port=1  Side=Left
  connections:
  Solid/RConn1 -- ReferenceFrame/RConn1 -- F/RConn1

== system QuadRotor_PID_Simulink3d/quadSimulation/Plant_Quad_Base/Quad_6Dof/QuadRotor/P3/MotorC/Helice_1_RIGID ==
  ReferenceFrame : sm_lib/Frames and Transforms/Reference Frame  BlockFunction=simmechanics.library.frames_transforms.reference_frame
  Solid : sm_lib/Body Elements/Solid  InertiaType=Custom  Mass=0.00049709299999999999  MassUnits=kg  CenterOfMass=[0 0 -0.00012752400000000001]  CenterOfMassUnits=mm  MomentsOfInertia=[0.0011848399999999999 0.31476899999999997 0.31557499999999999]  MomentsOfInertiaUnits=kg*mm^2  ProductsOfInertia=[0 0 -7.1669699999999998e-06]  ProductsOfInertiaUnits=kg*mm^2  DensityBased=on  Density=1000  DensityUnits=kg/(m^3)  GraphicType=FromGeometry  MarkerShape=Sphere  MarkerSize=10  MarkerSizeUnits=m  GraphicVisPropType=SimpleVisualProperties  GraphicDiffuseColor=[1 1 1]  GraphicSpecularColor=[0.5 0.5 0.5 1.0]  GraphicAmbientColor=[0.15 0.15 0.15 1.0]  GraphicEmissiveColor=[0.0 0.0 0.0 1.0]  GraphicShininess=75  GraphicOpacity=1  GeometryShape=FromFile  RectangleSize=[1 1]  RectangleSizeUnits=m  BrickDimensions=[1 1 1]  BrickDimensionUnits=m  CylinderRadius=1  CylinderRadiusUnits=m  CylinderLength=1  CylinderLengthUnits=m  SphereRadius=1  SphereRadiusUnits=m  EllipsoidRadii=[1 1 1]  EllipsoidRadiiUnits=m  ExtrusionCrossSection=[1 1; -1 1; -1 -1; 1 -1]  ExtrusionCrossSectionUnits=m  ExtrusionLength=1  ExtrusionLengthUnits=m  PolygonNumSides=3  PolygonOuterRadius=1  PolygonOuterRadiusUnits=m  ExtGeomFileType=STL  ExtGeomFileName=Helice_Valor predeterminado_sldprt.STL  ExtGeomFileUnits=mm  RevolutionCrossSection=[1 1; 1 -1; 2 -1; 2 1]  RevolutionCrossSectionUnits=m  RevolutionExtent=Full  RevolutionAngle=180  RevolutionAngleUnits=deg  BlockFunction=simmechanics.library.body_elements.solid
  F : PMIOPort  Port=1  Side=Left
  connections:
  Solid/RConn1 -- ReferenceFrame/RConn1 -- F/RConn1

== system QuadRotor_PID_Simulink3d/quadSimulation/Plant_Quad_Base/Quad_6Dof/QuadRotor/P3/MotorC/x18_11_2000kv_Micro_Brushless_1_RIGID ==
  ReferenceFrame : sm_lib/Frames and Transforms/Reference Frame  BlockFunction=simmechanics.library.frames_transforms.reference_frame
  Solid : sm_lib/Body Elements/Solid  InertiaType=Custom  Mass=10  MassUnits=g  CenterOfMass=[0 12.8438 0]  CenterOfMassUnits=mm  MomentsOfInertia=[0.43731300000000001 0.28562900000000002 0.43731300000000001]  MomentsOfInertiaUnits=kg*mm^2  ProductsOfInertia=[0 0 0]  ProductsOfInertiaUnits=kg*mm^2  DensityBased=on  Density=1000  DensityUnits=kg/(m^3)  GraphicType=FromGeometry  MarkerShape=Sphere  MarkerSize=10  MarkerSizeUnits=m  GraphicVisPropType=SimpleVisualProperties  GraphicDiffuseColor=[0.894118 0.913725 0.929412]  GraphicSpecularColor=[0.5 0.5 0.5 1.0]  GraphicAmbientColor=[0.15 0.15 0.15 1.0]  GraphicEmissiveColor=[0.0 0.0 0.0 1.0]  GraphicShininess=75  GraphicOpacity=1  GeometryShape=FromFile  RectangleSize=[1 1]  RectangleSizeUnits=m  BrickDimensions=[1 1 1]  BrickDimensionUnits=m  CylinderRadius=1  CylinderRadiusUnits=m  CylinderLength=1  CylinderLengthUnits=m  SphereRadius=1  SphereRadiusUnits=m  EllipsoidRadii=[1 1 1]  EllipsoidRadiiUnits=m  ExtrusionCrossSection=[1 1; -1 1; -1 -1; 1 -1]  ExtrusionCrossSectionUnits=m  ExtrusionLength=1  ExtrusionLengthUnits=m  PolygonNumSides=3  PolygonOuterRadius=1  PolygonOuterRadiusUnits=m  ExtGeomFileType=STL  ExtGeomFileName=18-11 2000kv Micro Brushless_Valor predeterminado_sldprt.STL  ExtGeomFileUnits=mm  RevolutionCrossSection=[1 1; 1 -1; 2 -1; 2 1]  RevolutionCrossSectionUnits=m  RevolutionExtent=Full  RevolutionAngle=180  RevolutionAngleUnits=deg  BlockFunction=simmechanics.library.body_elements.solid
  F : PMIOPort  Port=1  Side=Left
  connections:
  Solid/RConn1 -- ReferenceFrame/RConn1 -- F/RConn1

== system QuadRotor_PID_Simulink3d/quadSimulation/Plant_Quad_Base/Quad_6Dof/QuadRotor/P4/MotorD/Helice_1_RIGID ==
  ReferenceFrame : sm_lib/Frames and Transforms/Reference Frame  BlockFunction=simmechanics.library.frames_transforms.reference_frame
  Solid : sm_lib/Body Elements/Solid  InertiaType=Custom  Mass=0.00049709299999999999  MassUnits=kg  CenterOfMass=[0 0 -0.00012752400000000001]  CenterOfMassUnits=mm  MomentsOfInertia=[0.0011848399999999999 0.31476899999999997 0.31557499999999999]  MomentsOfInertiaUnits=kg*mm^2  ProductsOfInertia=[0 0 -7.1669699999999998e-06]  ProductsOfInertiaUnits=kg*mm^2  DensityBased=on  Density=1000  DensityUnits=kg/(m^3)  GraphicType=FromGeometry  MarkerShape=Sphere  MarkerSize=10  MarkerSizeUnits=m  GraphicVisPropType=SimpleVisualProperties  GraphicDiffuseColor=[1 1 1]  GraphicSpecularColor=[0.5 0.5 0.5 1.0]  GraphicAmbientColor=[0.15 0.15 0.15 1.0]  GraphicEmissiveColor=[0.0 0.0 0.0 1.0]  GraphicShininess=75  GraphicOpacity=1  GeometryShape=FromFile  RectangleSize=[1 1]  RectangleSizeUnits=m  BrickDimensions=[1 1 1]  BrickDimensionUnits=m  CylinderRadius=1  CylinderRadiusUnits=m  CylinderLength=1  CylinderLengthUnits=m  SphereRadius=1  SphereRadiusUnits=m  EllipsoidRadii=[1 1 1]  EllipsoidRadiiUnits=m  ExtrusionCrossSection=[1 1; -1 1; -1 -1; 1 -1]  ExtrusionCrossSectionUnits=m  ExtrusionLength=1  ExtrusionLengthUnits=m  PolygonNumSides=3  PolygonOuterRadius=1  PolygonOuterRadiusUnits=m  ExtGeomFileType=STL  ExtGeomFileName=Helice_Valor predeterminado_sldprt.STL  ExtGeomFileUnits=mm  RevolutionCrossSection=[1 1; 1 -1; 2 -1; 2 1]  RevolutionCrossSectionUnits=m  RevolutionExtent=Full  RevolutionAngle=180  RevolutionAngleUnits=deg  BlockFunction=simmechanics.library.body_elements.solid
  F : PMIOPort  Port=1  Side=Left
  connections:
  Solid/RConn1 -- ReferenceFrame/RConn1 -- F/RConn1

== system QuadRotor_PID_Simulink3d/quadSimulation/Plant_Quad_Base/Quad_6Dof/QuadRotor/P4/MotorD/x18_11_2000kv_Micro_Brushless_1_RIGID ==
  ReferenceFrame : sm_lib/Frames and Transforms/Reference Frame  BlockFunction=simmechanics.library.frames_transforms.reference_frame
  Solid : sm_lib/Body Elements/Solid  InertiaType=Custom  Mass=10  MassUnits=g  CenterOfMass=[0 12.8438 0]  CenterOfMassUnits=mm  MomentsOfInertia=[0.43731300000000001 0.28562900000000002 0.43731300000000001]  MomentsOfInertiaUnits=kg*mm^2  ProductsOfInertia=[0 0 0]  ProductsOfInertiaUnits=kg*mm^2  DensityBased=on  Density=1000  DensityUnits=kg/(m^3)  GraphicType=FromGeometry  MarkerShape=Sphere  MarkerSize=10  MarkerSizeUnits=m  GraphicVisPropType=SimpleVisualProperties  GraphicDiffuseColor=[0.894118 0.913725 0.929412]  GraphicSpecularColor=[0.5 0.5 0.5 1.0]  GraphicAmbientColor=[0.15 0.15 0.15 1.0]  GraphicEmissiveColor=[0.0 0.0 0.0 1.0]  GraphicShininess=75  GraphicOpacity=1  GeometryShape=FromFile  RectangleSize=[1 1]  RectangleSizeUnits=m  BrickDimensions=[1 1 1]  BrickDimensionUnits=m  CylinderRadius=1  CylinderRadiusUnits=m  CylinderLength=1  CylinderLengthUnits=m  SphereRadius=1  SphereRadiusUnits=m  EllipsoidRadii=[1 1 1]  EllipsoidRadiiUnits=m  ExtrusionCrossSection=[1 1; -1 1; -1 -1; 1 -1]  ExtrusionCrossSectionUnits=m  ExtrusionLength=1  ExtrusionLengthUnits=m  PolygonNumSides=3  PolygonOuterRadius=1  PolygonOuterRadiusUnits=m  ExtGeomFileType=STL  ExtGeomFileName=18-11 2000kv Micro Brushless_Valor predeterminado_sldprt.STL  ExtGeomFileUnits=mm  RevolutionCrossSection=[1 1; 1 -1; 2 -1; 2 1]  RevolutionCrossSectionUnits=m  RevolutionExtent=Full  RevolutionAngle=180  RevolutionAngleUnits=deg  BlockFunction=simmechanics.library.body_elements.solid
  F : PMIOPort  Port=1  Side=Left
  connections:
  Solid/RConn1 -- ReferenceFrame/RConn1 -- F/RConn1

== system QuadRotor_PID_Simulink3d/quadSimulation/Plant_Quad_Base/Quad_Altitude/QuadRotor/P1/MotorB/Helice_1_RIGID ==
  ReferenceFrame : sm_lib/Frames and Transforms/Reference Frame  BlockFunction=simmechanics.library.frames_transforms.reference_frame
  Solid : sm_lib/Body Elements/Solid  InertiaType=Custom  Mass=0.00049709299999999999  MassUnits=kg  CenterOfMass=[0 0 -0.00012752400000000001]  CenterOfMassUnits=mm  MomentsOfInertia=[0.0011848399999999999 0.31476899999999997 0.31557499999999999]  MomentsOfInertiaUnits=kg*mm^2  ProductsOfInertia=[0 0 -7.1669699999999998e-06]  ProductsOfInertiaUnits=kg*mm^2  DensityBased=on  Density=1000  DensityUnits=kg/(m^3)  GraphicType=FromGeometry  MarkerShape=Sphere  MarkerSize=10  MarkerSizeUnits=m  GraphicVisPropType=SimpleVisualProperties  GraphicDiffuseColor=[1 1 1]  GraphicSpecularColor=[0.5 0.5 0.5 1.0]  GraphicAmbientColor=[0.15 0.15 0.15 1.0]  GraphicEmissiveColor=[0.0 0.0 0.0 1.0]  GraphicShininess=75  GraphicOpacity=1  GeometryShape=FromFile  RectangleSize=[1 1]  RectangleSizeUnits=m  BrickDimensions=[1 1 1]  BrickDimensionUnits=m  CylinderRadius=1  CylinderRadiusUnits=m  CylinderLength=1  CylinderLengthUnits=m  SphereRadius=1  SphereRadiusUnits=m  EllipsoidRadii=[1 1 1]  EllipsoidRadiiUnits=m  ExtrusionCrossSection=[1 1; -1 1; -1 -1; 1 -1]  ExtrusionCrossSectionUnits=m  ExtrusionLength=1  ExtrusionLengthUnits=m  PolygonNumSides=3  PolygonOuterRadius=1  PolygonOuterRadiusUnits=m  ExtGeomFileType=STL  ExtGeomFileName=Helice_Valor predeterminado_sldprt.STL  ExtGeomFileUnits=mm  RevolutionCrossSection=[1 1; 1 -1; 2 -1; 2 1]  RevolutionCrossSectionUnits=m  RevolutionExtent=Full  RevolutionAngle=180  RevolutionAngleUnits=deg  BlockFunction=simmechanics.library.body_elements.solid
  F : PMIOPort  Port=1  Side=Left
  connections:
  Solid/RConn1 -- ReferenceFrame/RConn1 -- F/RConn1

== system QuadRotor_PID_Simulink3d/quadSimulation/Plant_Quad_Base/Quad_Altitude/QuadRotor/P1/MotorB/x18_11_2000kv_Micro_Brushless_1_RIGID ==
  ReferenceFrame : sm_lib/Frames and Transforms/Reference Frame  BlockFunction=simmechanics.library.frames_transforms.reference_frame
  Solid : sm_lib/Body Elements/Solid  InertiaType=Custom  Mass=10  MassUnits=g  CenterOfMass=[0 12.8438 0]  CenterOfMassUnits=mm  MomentsOfInertia=[0.43731300000000001 0.28562900000000002 0.43731300000000001]  MomentsOfInertiaUnits=kg*mm^2  ProductsOfInertia=[0 0 0]  ProductsOfInertiaUnits=kg*mm^2  DensityBased=on  Density=1000  DensityUnits=kg/(m^3)  GraphicType=FromGeometry  MarkerShape=Sphere  MarkerSize=10  MarkerSizeUnits=m  GraphicVisPropType=SimpleVisualProperties  GraphicDiffuseColor=[0.894118 0.913725 0.929412]  GraphicSpecularColor=[0.5 0.5 0.5 1.0]  GraphicAmbientColor=[0.15 0.15 0.15 1.0]  GraphicEmissiveColor=[0.0 0.0 0.0 1.0]  GraphicShininess=75  GraphicOpacity=1  GeometryShape=FromFile  RectangleSize=[1 1]  RectangleSizeUnits=m  BrickDimensions=[1 1 1]  BrickDimensionUnits=m  CylinderRadius=1  CylinderRadiusUnits=m  CylinderLength=1  CylinderLengthUnits=m  SphereRadius=1  SphereRadiusUnits=m  EllipsoidRadii=[1 1 1]  EllipsoidRadiiUnits=m  ExtrusionCrossSection=[1 1; -1 1; -1 -1; 1 -1]  ExtrusionCrossSectionUnits=m  ExtrusionLength=1  ExtrusionLengthUnits=m  PolygonNumSides=3  PolygonOuterRadius=1  PolygonOuterRadiusUnits=m  ExtGeomFileType=STL  ExtGeomFileName=18-11 2000kv Micro Brushless_Valor predeterminado_sldprt.STL  ExtGeomFileUnits=mm  RevolutionCrossSection=[1 1; 1 -1; 2 -1; 2 1]  RevolutionCrossSectionUnits=m  RevolutionExtent=Full  RevolutionAngle=180  RevolutionAngleUnits=deg  BlockFunction=simmechanics.library.body_elements.solid
  F : PMIOPort  Port=1  Side=Left
  connections:
  Solid/RConn1 -- ReferenceFrame/RConn1 -- F/RConn1
